simulink model "DC_Machine_Characteristics"  (R2023a)
settings: Solver=VariableStepAuto  StartTime=0.0  StopTime=4  RelTol=1e-3
values from neighbouring files (symbols this model uses):
  bm = 0.01    [DC_Machien_Characteristics.m]
  J = 0.0167    [DC_Machien_Characteristics.m]
  Ke = 0.8    [DC_Machien_Characteristics.m]
  L = 0.003    [DC_Machien_Characteristics.m]
  R = 0.5    [DC_Machien_Characteristics.m]
settings Model: Creator=koush  LastModifiedBy=koush

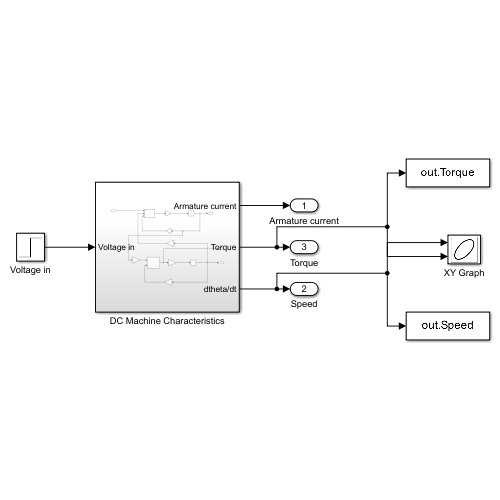
[thumbnail: Simulink's stored preview of the top-level diagram]
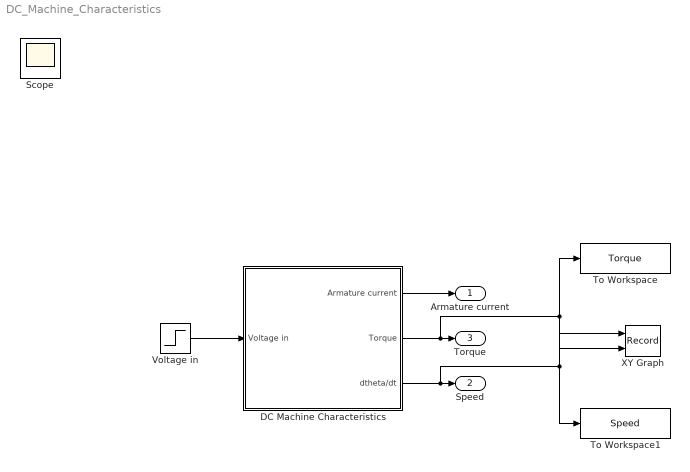
== system DC_Machine_Characteristics ==
  DC Machine Characteristics : Subsystem
  To Workspace : ToWorkspace  VariableName=Torque  SampleTime=-1
  To Workspace1 : ToWorkspace  VariableName=Speed  SampleTime=-1
  Voltage in : Step  After=220  SampleTime=0.001
  XY Graph : Record  FileSettingsInternal="{\"entries\":[{\"content\":{\"excelSettings\":{\"content\":{},\"type\":\"Streamout.ExcelSettings\"}},\"type\":\"Streamout.FileSettingStorage\",\"uuid\":\"\"}],\"packageUris\":[\"http:\\/\\/schema.mathworks.com\\/mf0\\/streamout_blocks\\/R2020a\"],\"version\":\"1.0\"}"  Layout=[1 1]  SignalsInternal="{\"entries\":[{\"content\":{\"signals\":[{\"content\":{\"blockPath\":[],\"dimensions\":[1],\"domain\":\"\",\"lineColor\":\"#a2142f\",\"plots\":[1],\"port\":1,\"sid\":[\"\"],\"signalID\":13064,\"signalName\":\"DC Machine Characteristics:3\"},\"type\":\"RecordBlkView.Signal\",\"uuid\":\"\"},{\"content\":{\"blockPath\":[],\"dimensions\":[1],\"domain\":\"\",\"lineColor\":\"#139fff\",\"plots\":[1],\"port\":2,\"sid\":[\"\"],\"signalID\":13068,\"signalName\":\"DC Machine Characteristics:2\"},\"type\":\"RecordBlkView.Signal\",\"uuid\":\"\"}]},\"type\":\"RecordBlkView.InputSignals\",\"uuid\":\"\"}],\"packageUris\":[\"http:\\/\\/schema.mathworks.com\\/mf0\\/streamout_blocks\\/R2020a\"],\"version\":\"1.0\"}"  VisualizationBindings="{\"xyplotplugin\":{\"info\":[{\"series\":[{\"bindingParametersList\":[{\"parameter\":\"X-Axis\",\"signalID\":13064,\"signalName\":\"DC Machine Characteristics:3\"},{\"parameter\":\"Y-Axis\",\"signalID\":13068,\"signalName\":\"DC Machine Characteristics:2\"}],\"seriesID\":44112}],\"subplotID\":1}]}}"  CompatibilityTag=XY
  Armature current : Outport
  Speed : Outport  Port=2
  Torque : Outport  Port=3
  Scope : Scope
  wires:
  Voltage in/1 -> DC Machine Characteristics/1(Voltage in)
  DC Machine Characteristics/1(Armature current) -> Armature current/1
  DC Machine Characteristics/2(Torque) -> To Workspace/1, XY Graph/2, Torque/1
  DC Machine Characteristics/3(dtheta/dt) -> To Workspace1/1, XY Graph/1, Speed/1

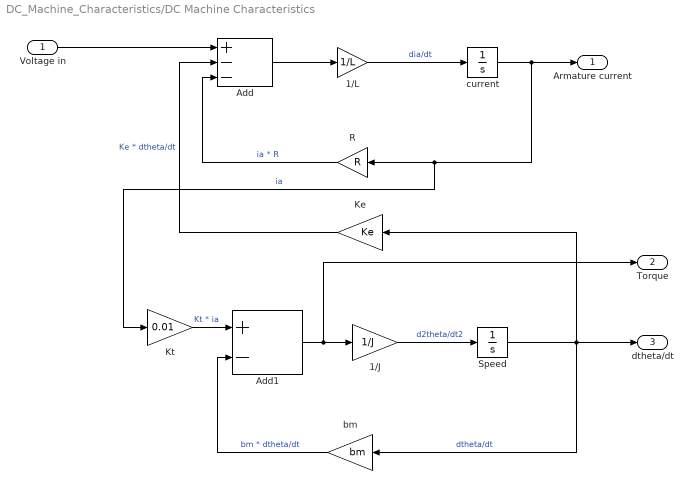
== system DC_Machine_Characteristics/DC Machine Characteristics ==
  Voltage in : Inport
  1/J : Gain  Gain=1/J
  1/L : Gain  Gain=1/L
  Add : Sum  Inputs=+--
  Add1 : Sum  Inputs=+-
  Ke : Gain  Gain=Ke
  Kt : Gain  Gain=0.01
  R : Gain  Gain=R
  Speed : Integrator
  bm : Gain  Gain=bm
  current : Integrator
  Armature current : Outport
  Torque : Outport  Port=2
  dtheta/dt : Outport  Port=3
  wires:
  Ke/1 -> Add/2  "Ke * dtheta/dt"
  Add1/1 -> Torque/1, 1/J/1
  bm/1 -> Add1/2  "bm * dtheta/dt"
  current/1 -> Armature current/1, Kt/1, R/1  "ia"
  Speed/1 -> dtheta/dt/1, bm/1, Ke/1  "dtheta/dt"
  Add/1 -> 1/L/1
  R/1 -> Add/3  "ia * R"
  1/L/1 -> current/1  "dia/dt"
  1/J/1 -> Speed/1  "d2theta/dt2"
  Kt/1 -> Add1/1  "Kt * ia"
  Voltage in/1 -> Add/1
